simulink model "kinf"  (R2016b)
settings: Solver=VariableStepAuto  StartTime=0.0  StopTime=10.0  RelTol=1e-3
values from neighbouring files (symbols this model uses):
  A = [-Ra1/La1     0            -Kb1/(r*La1)          -Kb1*l/(2*r*La1) ... (first row only)    [lqgfin.m]
  B = [1/La1 0 ... (first row only)    [lqgfin.m]
  C = [0    0    1/r  l/(2*r) ... (first row only)    [lqgfin.m]
  Cx = [0 0 1 0 0 0;0 0 0 1 0 0;0 0 0 0 1 0; 0 0 0 0 0 1]    [lqgfin.m]
  Cy = [1 0 0 0 0 0;0 1 0 0 0 0]    [lqgfin.m]
  l = 0.21    [lqgfin.m]
  r = 0.13/2    (= 0.065)    [lqgfin.m]
undefined symbols (not defined in the file or in its folder): An, Bn, Cn, Dn, K_lqi
libraries: Controllers x2, DiffSteer_model x1
settings Model: Creator=Hamza  LastModifiedBy=Hamza

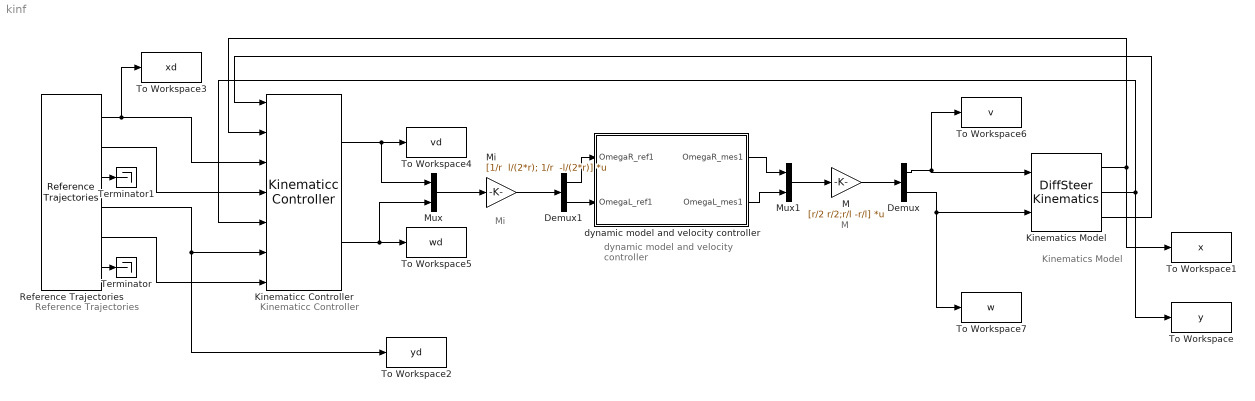
== system kinf ==
  note: M
  note: Kinematics
      | Model
  note: dynamic model
      | and velocity controller
  note: Kinematicc
      | Controller
  note: Reference
      | Trajectories
  note: Mi
  " Kinematics Model" : DiffSteer_model/DiffSteer Kinematics  x0=[0, 0, 0]  a=0.18  umax=0.65  wmax=6.2  dumax=5  dwmax=5
  Demux : Demux  Outputs=2
  Demux1 : Demux  Outputs=2
  Kinematicc Controller : Controllers/Kinematicc Controller  kx=1  ky=1  lx=0.25  ly=0.25  a=0
      link override 1//a: Gain=1/0.18
  M : Gain  Gain=[r/2 r/2;r/l -r/l]  Multiplication=Matrix(K*u)
  Mi : Gain  Gain="[1/r  l/(2*r); 1/r  -l/(2*r)]"  Multiplication=Matrix(K*u)
  Mux : Mux  Inputs=2
  Mux1 : Mux  Inputs=2
  Reference Trajectories : Controllers/Reference Trajectories  trajectory_type=2  wf=0.2  raio_ref_1=1  delta_raio=-0.2  t_delta_raio=100  xd=[2.5, 2.5]
  Terminator : Terminator
  Terminator1 : Terminator
  To Workspace : ToWorkspace  VariableName=y  SampleTime=-1
  To Workspace1 : ToWorkspace  VariableName=x  SampleTime=-1
  To Workspace2 : ToWorkspace  VariableName=yd  SampleTime=-1
  To Workspace3 : ToWorkspace  VariableName=xd  SampleTime=-1
  To Workspace4 : ToWorkspace  VariableName=vd  SampleTime=-1
  To Workspace5 : ToWorkspace  VariableName=wd  SampleTime=-1
  To Workspace6 : ToWorkspace  VariableName=v  SampleTime=-1
  To Workspace7 : ToWorkspace  VariableName=w  SampleTime=-1
  dynamic model and velocity controller : Subsystem
  wires:
  Reference Trajectories/1 -> Kinematicc Controller/3, To Workspace3/1
  Reference Trajectories/2 -> Kinematicc Controller/4
  Reference Trajectories/4 -> Kinematicc Controller/6, To Workspace2/1
  Reference Trajectories/5 -> Kinematicc Controller/7
  " Kinematics Model"/1 -> Kinematicc Controller/2, To Workspace1/1
  " Kinematics Model"/2 -> Kinematicc Controller/5, To Workspace/1
  " Kinematics Model"/3 -> Kinematicc Controller/1
  Reference Trajectories/3 -> Terminator1/1
  Reference Trajectories/6 -> Terminator/1
  Mux1/1 -> M/1
  Mux/1 -> Mi/1
  M/1 -> Demux/1
  Mi/1 -> Demux1/1
  Demux1/1 -> dynamic model and velocity controller/1(OmegaR_ref1)
  Demux1/2 -> dynamic model and velocity controller/2(OmegaL_ref1)
  dynamic model and velocity controller/1(OmegaR_mes1) -> Mux1/1
  dynamic model and velocity controller/2(OmegaL_mes1) -> Mux1/2
  Kinematicc Controller/2 -> To Workspace5/1, Mux/2
  Kinematicc Controller/1 -> To Workspace4/1, Mux/1
  Demux/1 -> " Kinematics Model"/1, To Workspace6/1
  Demux/2 -> To Workspace7/1, " Kinematics Model"/2

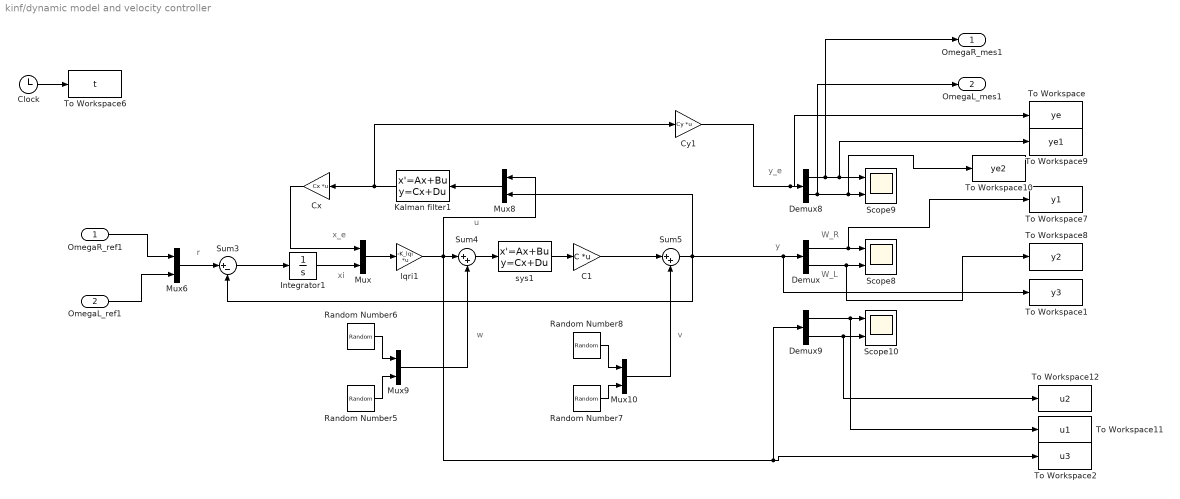
== system kinf/dynamic model and velocity controller ==
  note: W_R
  note: r
  note: y_e
  note: xi
  note: x_e
  note: u
  note: y
  note: W_L
  note: w
  note: v
  OmegaR_ref1 : Inport
  OmegaL_ref1 : Inport  Port=2
  "  Cx" : Gain  Gain=Cx  Multiplication=Matrix(K*u)
  C1 : Gain  Gain=C  Multiplication=Matrix(K*u)
  Clock : Clock
  Cy1 : Gain  Gain=Cy  Multiplication=Matrix(K*u)
  Demux : Demux  Outputs=2
  Demux8 : Demux  Outputs=2
  Demux9 : Demux  Outputs=2
  Integrator1 : Integrator
  Kalman filter1 : StateSpace  A=An  B=Bn  C=Cn  D=Dn  X0=0
  Mux{,6,8..10} (5 alike) : Mux  Inputs=2
  Random Number5 : RandomNumber  Variance=0.1  Seed=40  SampleTime=0.01
  Random Number6 : RandomNumber  Variance=0.1  Seed=25  SampleTime=0.01
  Random Number7 : RandomNumber  Variance=0.1  Seed=30  SampleTime=0.01
  Random Number8 : RandomNumber  Variance=0.1  Seed=20  SampleTime=0.01
  Scope10 : Scope  NumInputPorts=2
  Scope8 : Scope  NumInputPorts=2
  Scope9 : Scope  NumInputPorts=2
  Sum3 : Sum  Inputs=|+-
  Sum4 : Sum  Inputs=|++
  Sum5 : Sum  Inputs=|++
  To Workspace : ToWorkspace  VariableName=ye  SampleTime=-1
  To Workspace1 : ToWorkspace  VariableName=y3  SampleTime=-1
  To Workspace10 : ToWorkspace  VariableName=ye2  SampleTime=-1
  To Workspace11 : ToWorkspace  VariableName=u1  SampleTime=-1
  To Workspace12 : ToWorkspace  VariableName=u2  SampleTime=-1
  To Workspace2 : ToWorkspace  VariableName=u3  SampleTime=-1
  To Workspace6 : ToWorkspace  VariableName=t  SampleTime=-1
  To Workspace7 : ToWorkspace  VariableName=y1  SampleTime=-1
  To Workspace8 : ToWorkspace  VariableName=y2  SampleTime=-1
  To Workspace9 : ToWorkspace  VariableName=ye1  SampleTime=-1
  lqri1 : Gain  Gain=-K_lqi  Multiplication=Matrix(K*u)
  sys1 : StateSpace  A=A  B=B  C=eye(4)  D=zeros(4,2)  X0=0
  OmegaR_mes1 : Outport
  OmegaL_mes1 : Outport  Port=2
  wires:
  Sum3/1 -> Integrator1/1
  Integrator1/1 -> Mux/2
  sys1/1 -> C1/1
  Mux/1 -> lqri1/1
  OmegaL_ref1/1 -> Mux6/2
  OmegaR_ref1/1 -> Mux6/1
  Mux6/1 -> Sum3/1
  Demux/1 -> To Workspace7/1, Scope8/1
  Demux/2 -> To Workspace8/1, Scope8/2
  Mux8/1 -> Kalman filter1/1
  Kalman filter1/1 -> Cy1/1, "  Cx"/1
  Random Number6/1 -> Mux9/1
  Random Number5/1 -> Mux9/2
  Random Number8/1 -> Mux10/1
  Random Number7/1 -> Mux10/2
  Sum5/1 -> Mux8/2, To Workspace1/1, Demux/1, Sum3/2
  Demux8/1 -> OmegaR_mes1/1, To Workspace9/1, Scope9/1
  Demux8/2 -> OmegaL_mes1/1, To Workspace10/1, Scope9/2
  Cy1/1 -> To Workspace/1, Demux8/1
  Sum4/1 -> sys1/1
  Demux9/1 -> To Workspace11/1, Scope10/1
  Demux9/2 -> To Workspace12/1, Scope10/2
  lqri1/1 -> Mux8/1, Demux9/1, To Workspace2/1, Sum4/1
  C1/1 -> Sum5/1
  Clock/1 -> To Workspace6/1
  Mux9/1 -> Sum4/2
  Mux10/1 -> Sum5/2
  "  Cx"/1 -> Mux/1
